simulink model "initControlHardware"  (R2022a)
settings: Solver=FixedStepAuto  StartTime=0.0  StopTime=1  FixedStep=T  RelTol=1e-3
values from neighbouring files (symbols this model uses):
  D = 1    [dataExperimentalOneVolt.mat]    (also in dataExperimentalThreeVolt.mat = 0.4; dataExperimentalTwoVolt.mat = 0.5; initExperimental.m = 0.4)
  g = 0.00157079632679    [dataExperimentalOneVolt.mat]    (also in dataExperimentalThreeVolt.mat; dataExperimentalTwoVolt.mat; initExperimental.m)
  H = 60    [dataControlHardware.mat]    (also in dataExperimentalOneVolt.mat = 1; dataExperimentalThreeVolt.mat = 3; dataExperimentalTwoVolt.mat = 2; initControlHardware.m)
  T = 0.001    [dataControlHardware.mat]    (also in dataExperimentalOneVolt.mat; dataExperimentalThreeVolt.mat; dataExperimentalTwoVolt.mat; initControlHardware.m)
undefined symbols (not defined in the file or in its folder): Humusoft, MF634
libraries: sldrtlib x2
settings Model: SimulationMode=external  ExtModeTrigDuration=100000  Creator=alexis_noriega  LastModifiedBy=alexis_noriega
settings DataIOCC: ReturnWorkspaceOutputs=off
settings HardwareCC: ProdBitPerLong=64  ProdHWDeviceType=Intel->x86-64 (Linux 64)
settings RTWCC: Description=Simulink Desktop Real-Time  SystemTargetFile=sldrt.tlc  TemplateMakefile=sldrt.tmf  RTWCompilerOptimization=on
settings CodeAppCC: MaxIdLength=95
settings SimulinkDesktopRealTimeCC: TargetLibSuffix=_sldrt.a  TargetPreCompLibLocation=C:\Program Files\MATLAB\R2022a\toolbox\sldrt\lib\win64

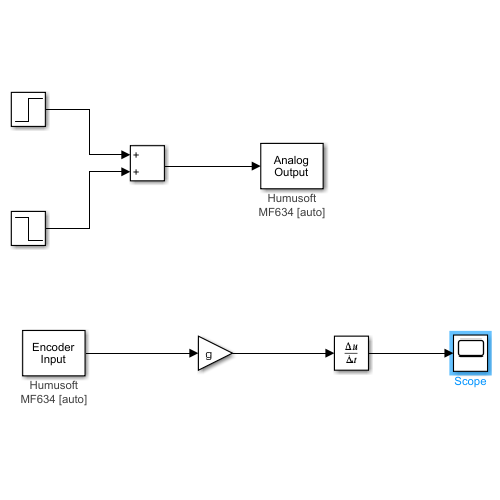
[thumbnail: Simulink's stored preview of the top-level diagram]
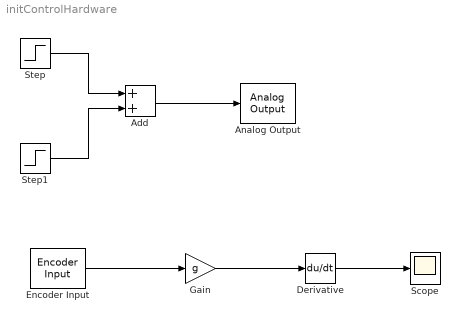
== system initControlHardware ==
  Add : Sum
  Analog Output : sldrtlib/Analog Output  SampleTime=T  MaxMissedTicks=10  ShowMissedTicks=off  YieldWhenWaiting=off  DrvName=Humusoft/MF634  DrvAddress=4294967295  DrvOptions=0  Channels=1  RangeMode=1  VoltRange=1  InitialValue=0  FinalValue=0
      settings: AttributesFormatString=Humusoft\nMF634 [auto]
  Derivative : Derivative
  Encoder Input : sldrtlib/Encoder Input  SampleTime=T  MaxMissedTicks=10  ShowMissedTicks=off  YieldWhenWaiting=off  DrvName=Humusoft/MF634  DrvAddress=4294967295  DrvOptions=0  Channels=1  QuadMode=3  IndexPulse=3  InputFilter=Inf  DataType=1
      settings: AttributesFormatString=Humusoft\nMF634 [auto]
  Gain : Gain  Gain=g
  Scope : Scope
  Step : Step  Time=0  After=H  SampleTime=T
  Step1 : Step  Time=D  After=-H  SampleTime=T
  wires:
  Step/1 -> Add/1
  Step1/1 -> Add/2
  Add/1 -> Analog Output/1
  Encoder Input/1 -> Gain/1
  Gain/1 -> Derivative/1
  Derivative/1 -> Scope/1
